simulink model "SuspSys_w_params"  (Simulink 7.7)
settings: Solver=ode45  StartTime=0.0  StopTime=5000  RelTol=1e-3
undefined symbols (not defined in the file): DamperDampingCoeffNspm, DamperSpringConstNpm, G, s, Suspension, suspension_lib, VehicleMassKg, WheelAssemblyMassKg, WheelDampingCoeffNspm, WheelSpringConstNpm
libraries: simulink x1
settings Model: Creator=jporter  LastModifiedBy=jporter

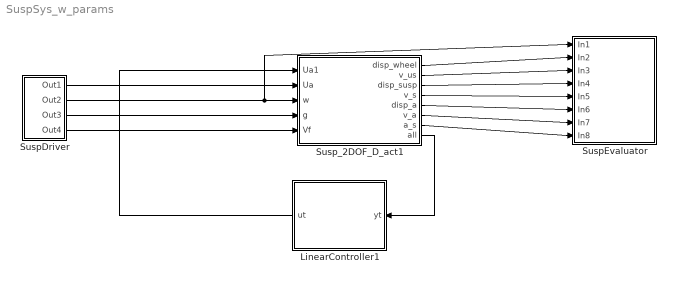
== system SuspSys_w_params ==
  LinearController1 : Subsystem
  SuspDriver : Subsystem
  SuspEvaluator : Subsystem
  Susp_2DOF_D_act1 : Subsystem  AncestorBlock=suspension_lib/Suspension:G(s)  mask{m_s=VehicleMassKg, k_s=DamperSpringConstNpm, b_s=DamperDampingCoeffNspm, m_us=WheelAssemblyMassKg, k_us=WheelSpringConstNpm, b_us=WheelDampingCoeffNspm, m_a=0, k_a=0, b_a=0}
      mask prompts: m_s "Sprung mass (kg)"; k_s "Sprung mass spring constant (N/m)"; b_s "Sprung mass damping coefficient (N s/m)"; m_us "Unsprung mass (kg)"; k_us "Unsprung mass spring constant (N/m)"; b_us "Unsprung mass damping coefficient (N s/m)"; m_a "Active Damper mass (kg)"; k_a "Active Damper spring constant (N/m)"; b_a "Active Damper damping coeff (N s/m)"
      mask init:
      | w = sqrt( k_us / m_us );
      | w_us = sqrt( k_us / m_us );
      | rho = m_s / m_us;
      | rho_a = 0;
      | g = 9.81; % m/s^2 gravitational acceleration
      | 
      | % m_s == 0 and m_us == 0 are not allowed
      | % Work around possible divide by zero when m_a == 0
      | %  build A by rows
      | A = [0 1 0 0 0 0]; 
      | A = [A; -(k_us/m_us) (-b_s/m_us)+(b_us/m_us) (k_s/m_us) (b_s/m_us) 0 0]; 
      | A = [A; 0 -1 0 1 0 0]; 
      | A = [A; 0 (b_s/m_s) -(k_s/m_s) (-b_s/m_s) 0 0];
      | if ( m_a ~= 0 )
      |   w_a = sqrt( k_a / m_a );
      |   eta_a = b_a / (2 * m_a * w_a);
      |   rho_a = m_us / m_a;  
      |   A = [A; 0 -1 0 0 0 1]; 
      |   A = [A; 0 2 * eta_a * w_a 0 0 -(w_a^2) -2 * eta_a * w_a];
      | else
      |   A = [A; 0 0 0 0 0 0];
      |   A = [A; 0 0 0 0 0 0];
      | end
      | 
      | A=-A;
      | 
      | % inputs: active damper control force, 
      | %   active suspension control force,
      | %   road velocity, gravity, and sprung mass force
      | B = [0 0 -1 0 0];
      | B = [B; rho rho -(b_us/m_us) -g 0];
      | B = [B; 0 0 0 0 0];
      | B = [B; 0 -1 0 0 -1];
      | B = [B; 0 0 0 0 0];
      | B = [B; -rho * rho_a 0 0 0 0];
      | 
      | 
      | % A = [0 1 0 0 0 0]; 
      | % A = [A; -(k_us/m_us)  (-b_a/m_us) 0 0 (k_a/m_us) (b_a/m_us)]; 
      | % A = [A; 0 -1 0 1 0 0]; 
      | % A = [A; 0 0 0 0 0 0];
      | % if ( m_a ~= 0 )
      | %   w_a = sqrt( k_a / m_a );
      | %   eta_a = b_a / (2 * m_a * w_a);
      | %   rho_a = m_us / m_a;  
      | %   A = [A; 0 -1 0 0 0 1]; 
      | %   A = [A; 0 2 * eta_a * w_a 0 0 -(w_a^2) -2 * eta_a * w_a];
      | % else
      | %   A = [A; 0 0 0 0 0 0];
      | %   A = [A; 0 0 0 0 0 0];
      | % end
  wires:
  SuspDriver/2(Out2) -> Susp_2DOF_D_act1/3(w), SuspEvaluator/1(In1)
  Susp_2DOF_D_act1/1(disp_wheel) -> SuspEvaluator/2(In2)
  Susp_2DOF_D_act1/2(v_us) -> SuspEvaluator/3(In3)
  Susp_2DOF_D_act1/3(disp_susp) -> SuspEvaluator/4(In4)
  Susp_2DOF_D_act1/4(v_s) -> SuspEvaluator/5(In5)
  Susp_2DOF_D_act1/5(disp_a) -> SuspEvaluator/6(In6)
  Susp_2DOF_D_act1/6(v_a) -> SuspEvaluator/7(In7)
  SuspDriver/1(Out1) -> Susp_2DOF_D_act1/2(Ua)
  SuspDriver/3(Out3) -> Susp_2DOF_D_act1/4(g)
  SuspDriver/4(Out4) -> Susp_2DOF_D_act1/5(Vf)
  Susp_2DOF_D_act1/7(a_s) -> SuspEvaluator/8(In8)
  Susp_2DOF_D_act1/8(all) -> LinearController1/1(yt)
  LinearController1/1(ut) -> Susp_2DOF_D_act1/1(Ua1)

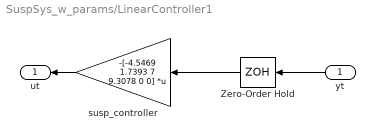
== system SuspSys_w_params/LinearController1 ==
  yt : Inport
  Zero-Order Hold : ZeroOrderHold  SampleTime=0.01
  susp_controller : Gain  Gain=-[-4.5469 1.7393 7 9.3078 0 0]  Multiplication=Matrix(K*u)
  ut : Outport
  wires:
  yt/1 -> Zero-Order Hold/1
  susp_controller/1 -> ut/1
  Zero-Order Hold/1 -> susp_controller/1

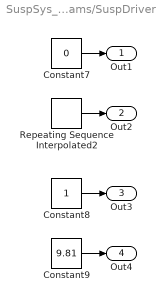
== system SuspSys_w_params/SuspDriver ==
  Constant7 : Constant  Value=0
  Constant8 : Constant
  Constant9 : Constant  Value=9.81
  Repeating Sequence Interpolated2 : simulink/Sources/Repeating Sequence Interpolated  SystemSampleTime=-1  OutValues=[0 0.5 0 -0.5 0 -0.5 0 0.5 0].'  TimeValues=[0 0.1 0.2 0.3 0.4 0.6 0.7 0.8 0.9].'  LookUpMeth=Interpolation-Use End Values  tsamp=0.01  OutMin=[]  OutMax=[]  OutDataTypeStr=double  OutputDataTypeScalingMode=double  OutDataType=fixdt(0,8)  OutScaling=2^-10
  Out1 : Outport
  Out2 : Outport  Port=2
  Out3 : Outport  Port=3
  Out4 : Outport  Port=4
  wires:
  Constant7/1 -> Out1/1
  Repeating Sequence Interpolated2/1 -> Out2/1
  Constant8/1 -> Out3/1
  Constant9/1 -> Out4/1

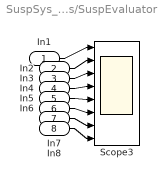
== system SuspSys_w_params/SuspEvaluator ==
  In1 : Inport
  In2 : Inport  Port=2
  In3 : Inport  Port=3
  In4 : Inport  Port=4
  In5 : Inport  Port=5
  In6 : Inport  Port=6
  In7 : Inport  Port=7
  In8 : Inport  Port=8
  Scope3 : Scope  NumInputPorts=8
      settings: YMin=-0.5~-0.5~-30~-0.9~-5~-5~-5~-5  YMax=0.5~0.5~30~0.3~5~5~5~5  SaveName=ScopeData2
  wires:
  In1/1 -> Scope3/1
  In2/1 -> Scope3/2
  In3/1 -> Scope3/3
  In4/1 -> Scope3/4
  In5/1 -> Scope3/5
  In6/1 -> Scope3/6
  In7/1 -> Scope3/7
  In8/1 -> Scope3/8

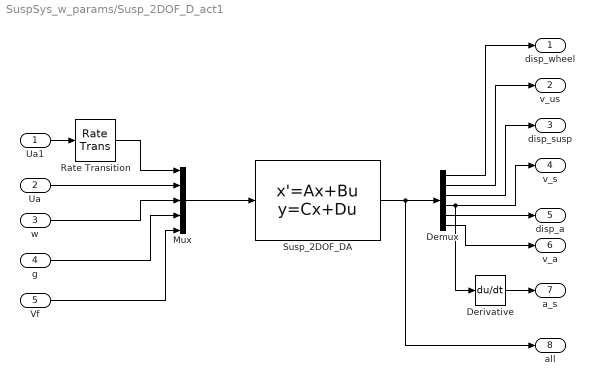
== system SuspSys_w_params/Susp_2DOF_D_act1 ==
  Ua1 : Inport
  Ua : Inport  Port=2
  w : Inport  Port=3
  g : Inport  Port=4
  Vf : Inport  Port=5
  Demux : Demux  Outputs=6
  Derivative : Derivative
  Mux : Mux  Inputs=5
  Rate Transition : RateTransition
  Susp_2DOF_DA : StateSpace  A=A  B=B  C=eye(6)  D=zeros(6,5)
  disp_wheel : Outport
  v_us : Outport  Port=2
  disp_susp : Outport  Port=3
  v_s : Outport  Port=4
  disp_a : Outport  Port=5
  v_a : Outport  Port=6
  a_s : Outport  Port=7
  all : Outport  Port=8
  wires:
  Ua/1 -> Mux/2
  w/1 -> Mux/3
  Mux/1 -> Susp_2DOF_DA/1
  Susp_2DOF_DA/1 -> Demux/1, all/1
  Demux/1 -> disp_wheel/1
  Demux/2 -> v_us/1
  Demux/3 -> disp_susp/1
  Demux/4 -> v_s/1, Derivative/1
  Demux/5 -> disp_a/1
  Demux/6 -> v_a/1
  g/1 -> Mux/4
  Vf/1 -> Mux/5
  Derivative/1 -> a_s/1
  Ua1/1 -> Rate Transition/1
  Rate Transition/1 -> Mux/1
